simulink model "gm_sampleModel61753_pp_45_1_sub"  (R2023b)
settings: Solver=VariableStepAuto  StartTime=0.0  StopTime=10.0  RelTol=1e-3
libraries: simulink x43
(part 2 of 2)

== system gm_sampleModel61753_pp_45_1_sub/Subsystem/cfblk4 ==
  note: U(k)
  note: Edge
  U : Inport  OutDataTypeStr=uint8  SampleTime=1
  Delay Input1 : UnitDelay  Description=Store in Global RAM  DisableCoverage=on  InitialCondition=vinit  SampleTime=-1  HasFrameUpgradeWarning=on
  FixPt Relational Operator : RelationalOperator  Operator=>  OutDataTypeStr=fixdt(0, 8)  ZeroCross=off  InputSameDT=off
  Nonpositive : Subsystem  mask(Compare To Zero){relop=<=, OutDataTypeStr=boolean, ZeroCross=off}
      mask prompts: relop "Simulink:masks:Operator_MP"; OutDataTypeStr "Simulink:masks:OutputDataType_MP"; ZeroCross "Simulink:masks:EnableZerocrossingDetection_MP"
      mask help: Simulink:masks:CompareToZero_MD
      mask init:
      | OutDataTypeStr = 'boolean';
      | ZeroCross = 'off';
      | blkName = 'sampleModel61753_pp_45_1_sub/Subsystem/cfblk4/Nonpositive';
      | relop = '<=';
      | setValue = 'boolean';
      mask TypeOptions relop: == | ~= | < | <= | >= | >
      mask TypeOptions OutDataTypeStr: Simulink:masks:uint8 | Simulink:masks:boolean
      mask Callback ZeroCross: sl('zeroCrossEnable', gcbh);
      mask Display: disp([relop,' 0'])
  Y : Outport  SampleTime=1
  wires:
  U/1 -> Nonpositive/1(u)
  Delay Input1/1 -> FixPt Relational Operator/2
  FixPt Relational Operator/1 -> Y/1
  Nonpositive/1(y) -> FixPt Relational Operator/1, Delay Input1/1

== system gm_sampleModel61753_pp_45_1_sub/Subsystem/cfblk41 ==
  emi_236 : Inport  OutDataTypeStr=uint8  PortDimensions=1  SampleTime=1
  Action Port : Inport  Port=2  OutDataTypeStr=boolean  SampleTime=1
  cfblk41 : MinMax
  cfblk41_out1bypassMux : MultiPortSwitch  DataPortOrder=Zero-based contiguous  Inputs=2  zeroidx=on  OutDataTypeStr=uint8  SampleTime=1  SaturateOnIntegerOverflow=off  InputSameDT=off
  emi_237_bypass : UnitDelay  InitialCondition="fi(0,0,8,0,\"hex\",\"00\")"  SampleTime=1
  emi_237 : Outport  SampleTime=1  InitialOutput=0
  wires:
  Action Port/1 -> cfblk41_out1bypassMux/1
  emi_236/1 -> cfblk41/1
  cfblk41/1 -> cfblk41_out1bypassMux/3
  cfblk41_out1bypassMux/1 -> emi_237_bypass/1, emi_237/1
  emi_237_bypass/1 -> cfblk41_out1bypassMux/2

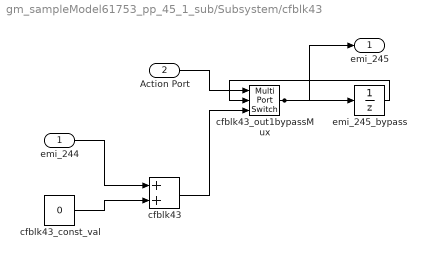
== system gm_sampleModel61753_pp_45_1_sub/Subsystem/cfblk43 ==
  emi_244 : Inport  OutDataTypeStr=uint8  PortDimensions=1  SampleTime=1
  Action Port : Inport  Port=2  OutDataTypeStr=boolean  SampleTime=1
  cfblk43 : Sum  OutDataTypeStr=uint8  AccumDataTypeStr=uint8  RndMeth=Nearest  SampleTime=1
  cfblk43_const_val : Constant  Value=0  VectorParams1D=off  OutDataTypeStr=uint8  SampleTime=1
  cfblk43_out1bypassMux : MultiPortSwitch  DataPortOrder=Zero-based contiguous  Inputs=2  zeroidx=on  OutDataTypeStr=uint8  SampleTime=1  SaturateOnIntegerOverflow=off  InputSameDT=off
  emi_245_bypass : UnitDelay  InitialCondition="fi(0,0,8,0,\"hex\",\"00\")"  SampleTime=1
  emi_245 : Outport  SampleTime=1  InitialOutput=0
  wires:
  Action Port/1 -> cfblk43_out1bypassMux/1
  emi_244/1 -> cfblk43/1
  cfblk43/1 -> cfblk43_out1bypassMux/3
  cfblk43_out1bypassMux/1 -> emi_245_bypass/1, emi_245/1
  emi_245_bypass/1 -> cfblk43_out1bypassMux/2
  cfblk43_const_val/1 -> cfblk43/2

== system gm_sampleModel61753_pp_45_1_sub/Subsystem/cfblk46 ==
  emi_252 : Inport  OutDataTypeStr=uint8  PortDimensions=1  SampleTime=1
  Action Port : Inport  Port=2  OutDataTypeStr=boolean  SampleTime=1
  cfblk46 : Sum  Inputs=+
  cfblk46_out1bypassMux : MultiPortSwitch  DataPortOrder=Zero-based contiguous  Inputs=2  zeroidx=on  OutDataTypeStr=uint8  SampleTime=1  SaturateOnIntegerOverflow=off  InputSameDT=off
  emi_253_bypass : UnitDelay  InitialCondition="fi(0,0,8,0,\"hex\",\"00\")"  SampleTime=1
  emi_253 : Outport  SampleTime=1  InitialOutput=0
  wires:
  Action Port/1 -> cfblk46_out1bypassMux/1
  emi_252/1 -> cfblk46/1
  cfblk46/1 -> cfblk46_out1bypassMux/3
  cfblk46_out1bypassMux/1 -> emi_253_bypass/1, emi_253/1
  emi_253_bypass/1 -> cfblk46_out1bypassMux/2

== system gm_sampleModel61753_pp_45_1_sub/Subsystem/cfblk48 ==
  emi_260 : Inport  OutDataTypeStr=uint8  PortDimensions=1  SampleTime=1
  Action Port : Inport  Port=2  OutDataTypeStr=boolean  SampleTime=1
  cfblk48 : Subsystem  mask(Real World Value Increment){}
      mask help: Simulink:masks:RealWorldValueIncrement_MD
      mask Display: disp('V++')
  cfblk48_out1bypassMux : MultiPortSwitch  DataPortOrder=Zero-based contiguous  Inputs=2  zeroidx=on  OutDataTypeStr=uint8  SampleTime=1  SaturateOnIntegerOverflow=off  InputSameDT=off
  emi_261_bypass : UnitDelay  InitialCondition="fi(0,0,8,0,\"hex\",\"00\")"  SampleTime=1
  emi_261 : Outport  SampleTime=1  InitialOutput=0
  wires:
  Action Port/1 -> cfblk48_out1bypassMux/1
  emi_260/1 -> cfblk48/1(u)
  cfblk48/1(y) -> cfblk48_out1bypassMux/3
  cfblk48_out1bypassMux/1 -> emi_261_bypass/1, emi_261/1
  emi_261_bypass/1 -> cfblk48_out1bypassMux/2

== system gm_sampleModel61753_pp_45_1_sub/Subsystem/cfblk50 ==
  emi_9 : Inport  OutDataTypeStr=uint8  PortDimensions=1  SampleTime=1
  Action Port : Inport  Port=2  OutDataTypeStr=boolean  SampleTime=1
  cfblk50 : Abs  SampleTime=1  OutDataTypeStr=uint8  SaturateOnIntegerOverflow=off
  cfblk50_out1bypassMux : MultiPortSwitch  DataPortOrder=Zero-based contiguous  Inputs=2  zeroidx=on  OutDataTypeStr=uint8  SampleTime=1  SaturateOnIntegerOverflow=off  InputSameDT=off
  emi_10_bypass : UnitDelay  InitialCondition="fi(0,0,8,0,\"hex\",\"00\")"  SampleTime=1
  emi_10 : Outport  SampleTime=1  InitialOutput=0
  wires:
  Action Port/1 -> cfblk50_out1bypassMux/1
  emi_9/1 -> cfblk50/1
  cfblk50/1 -> cfblk50_out1bypassMux/3
  cfblk50_out1bypassMux/1 -> emi_10_bypass/1, emi_10/1
  emi_10_bypass/1 -> cfblk50_out1bypassMux/2

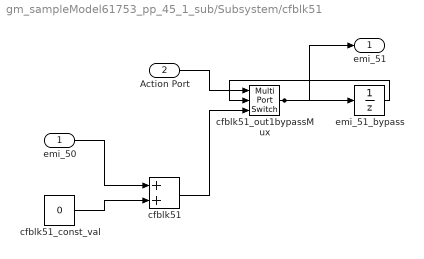
== system gm_sampleModel61753_pp_45_1_sub/Subsystem/cfblk51 ==
  emi_50 : Inport  OutDataTypeStr=uint8  PortDimensions=1  SampleTime=1
  Action Port : Inport  Port=2  OutDataTypeStr=boolean  SampleTime=1
  cfblk51 : Sum  OutDataTypeStr=uint8  AccumDataTypeStr=uint8  RndMeth=Nearest  SampleTime=1
  cfblk51_const_val : Constant  Value=0  VectorParams1D=off  OutDataTypeStr=uint8  SampleTime=1
  cfblk51_out1bypassMux : MultiPortSwitch  DataPortOrder=Zero-based contiguous  Inputs=2  zeroidx=on  OutDataTypeStr=uint8  SampleTime=1  SaturateOnIntegerOverflow=off  InputSameDT=off
  emi_51_bypass : UnitDelay  InitialCondition="fi(0,0,8,0,\"hex\",\"00\")"  SampleTime=1
  emi_51 : Outport  SampleTime=1  InitialOutput=0
  wires:
  Action Port/1 -> cfblk51_out1bypassMux/1
  emi_50/1 -> cfblk51/1
  cfblk51/1 -> cfblk51_out1bypassMux/3
  cfblk51_out1bypassMux/1 -> emi_51_bypass/1, emi_51/1
  emi_51_bypass/1 -> cfblk51_out1bypassMux/2
  cfblk51_const_val/1 -> cfblk51/2

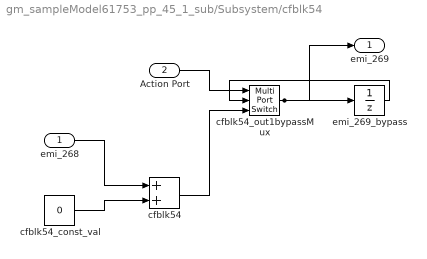
== system gm_sampleModel61753_pp_45_1_sub/Subsystem/cfblk54 ==
  emi_268 : Inport  OutDataTypeStr=uint8  PortDimensions=1  SampleTime=1
  Action Port : Inport  Port=2  OutDataTypeStr=boolean  SampleTime=1
  cfblk54 : Sum  OutDataTypeStr=uint8  AccumDataTypeStr=uint8  RndMeth=Nearest  SampleTime=1
  cfblk54_const_val : Constant  Value=0  VectorParams1D=off  OutDataTypeStr=uint8  SampleTime=1
  cfblk54_out1bypassMux : MultiPortSwitch  DataPortOrder=Zero-based contiguous  Inputs=2  zeroidx=on  OutDataTypeStr=uint8  SampleTime=1  SaturateOnIntegerOverflow=off  InputSameDT=off
  emi_269_bypass : UnitDelay  InitialCondition="fi(0,0,8,0,\"hex\",\"00\")"  SampleTime=1
  emi_269 : Outport  SampleTime=1  InitialOutput=0
  wires:
  Action Port/1 -> cfblk54_out1bypassMux/1
  emi_268/1 -> cfblk54/1
  cfblk54/1 -> cfblk54_out1bypassMux/3
  cfblk54_out1bypassMux/1 -> emi_269_bypass/1, emi_269/1
  emi_269_bypass/1 -> cfblk54_out1bypassMux/2
  cfblk54_const_val/1 -> cfblk54/2

== system gm_sampleModel61753_pp_45_1_sub/Subsystem/cfblk57 ==
  emi_276 : Inport  OutDataTypeStr=uint8  PortDimensions=1  SampleTime=1
  Action Port : Inport  Port=2  OutDataTypeStr=boolean  SampleTime=1
  cfblk57 : Signum  SampleTime=1
  cfblk57_out1bypassMux : MultiPortSwitch  DataPortOrder=Zero-based contiguous  Inputs=2  zeroidx=on  OutDataTypeStr=uint8  SampleTime=1  SaturateOnIntegerOverflow=off  InputSameDT=off
  emi_277_bypass : UnitDelay  InitialCondition="fi(0,0,8,0,\"hex\",\"00\")"  SampleTime=1
  emi_277 : Outport  SampleTime=1  InitialOutput=0
  wires:
  Action Port/1 -> cfblk57_out1bypassMux/1
  emi_276/1 -> cfblk57/1
  cfblk57/1 -> cfblk57_out1bypassMux/3
  cfblk57_out1bypassMux/1 -> emi_277_bypass/1, emi_277/1
  emi_277_bypass/1 -> cfblk57_out1bypassMux/2

== system gm_sampleModel61753_pp_45_1_sub/Subsystem/cfblk58 ==
  emi_284 : Inport  OutDataTypeStr=uint8  PortDimensions=1  SampleTime=1
  Action Port : Inport  Port=2  OutDataTypeStr=boolean  SampleTime=1
  cfblk58 : MinMax
  cfblk58_out1bypassMux : MultiPortSwitch  DataPortOrder=Zero-based contiguous  Inputs=2  zeroidx=on  OutDataTypeStr=uint8  SampleTime=1  SaturateOnIntegerOverflow=off  InputSameDT=off
  emi_285_bypass : UnitDelay  InitialCondition="fi(0,0,8,0,\"hex\",\"00\")"  SampleTime=1
  emi_285 : Outport  SampleTime=1  InitialOutput=0
  wires:
  Action Port/1 -> cfblk58_out1bypassMux/1
  emi_284/1 -> cfblk58/1
  cfblk58/1 -> cfblk58_out1bypassMux/3
  cfblk58_out1bypassMux/1 -> emi_285_bypass/1, emi_285/1
  emi_285_bypass/1 -> cfblk58_out1bypassMux/2

== system gm_sampleModel61753_pp_45_1_sub/Subsystem/cfblk62_inst ==
  in1 : Inport  OutDataTypeStr=uint8  SampleTime=1
  in2 : Inport  Port=2  OutDataTypeStr=uint8  SampleTime=1
  mul_cfblk62_dotp_mulcomp : Product  Inputs=**  OutDataTypeStr=uint8  SampleTime=1
  out1 : Outport  OutDataTypeStr=uint8  SampleTime=1
  wires:
  in1/1 -> mul_cfblk62_dotp_mulcomp/1
  in2/1 -> mul_cfblk62_dotp_mulcomp/2
  mul_cfblk62_dotp_mulcomp/1 -> out1/1

== system gm_sampleModel61753_pp_45_1_sub/Subsystem/cfblk65_inst ==
  in1 : Inport  OutDataTypeStr=uint8  SampleTime=1
  in2 : Inport  Port=2  OutDataTypeStr=uint8  SampleTime=1
  mul_cfblk65_dotp_mulcomp : Product  Inputs=**  OutDataTypeStr=uint8  SampleTime=1
  out1 : Outport  OutDataTypeStr=uint8  SampleTime=1
  wires:
  in1/1 -> mul_cfblk65_dotp_mulcomp/1
  in2/1 -> mul_cfblk65_dotp_mulcomp/2
  mul_cfblk65_dotp_mulcomp/1 -> out1/1

== system gm_sampleModel61753_pp_45_1_sub/Subsystem/cfblk69 ==
  emi_196 : Inport  OutDataTypeStr=uint8  PortDimensions=1  SampleTime=1
  Action Port : Inport  Port=2  OutDataTypeStr=boolean  SampleTime=1
  cfblk69 : Sum  Inputs=+
  cfblk69_out1bypassMux : MultiPortSwitch  DataPortOrder=Zero-based contiguous  Inputs=2  zeroidx=on  OutDataTypeStr=uint8  SampleTime=1  SaturateOnIntegerOverflow=off  InputSameDT=off
  emi_197_bypass : UnitDelay  InitialCondition="fi(0,0,8,0,\"hex\",\"00\")"  SampleTime=1
  emi_197 : Outport  SampleTime=1  InitialOutput=0
  wires:
  Action Port/1 -> cfblk69_out1bypassMux/1
  emi_196/1 -> cfblk69/1
  cfblk69/1 -> cfblk69_out1bypassMux/3
  cfblk69_out1bypassMux/1 -> emi_197_bypass/1, emi_197/1
  emi_197_bypass/1 -> cfblk69_out1bypassMux/2

== system gm_sampleModel61753_pp_45_1_sub/Subsystem/cfblk6_inst ==
  in1 : Inport  OutDataTypeStr=uint8  SampleTime=1
  in2 : Inport  Port=2  OutDataTypeStr=uint8  SampleTime=1
  mul_cfblk6_dotp_mulcomp : Product  Inputs=**  OutDataTypeStr=uint8  SampleTime=1
  out1 : Outport  OutDataTypeStr=uint8  SampleTime=1
  wires:
  in1/1 -> mul_cfblk6_dotp_mulcomp/1
  in2/1 -> mul_cfblk6_dotp_mulcomp/2
  mul_cfblk6_dotp_mulcomp/1 -> out1/1

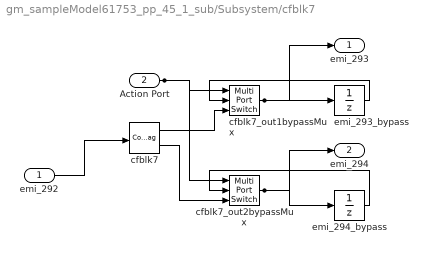
== system gm_sampleModel61753_pp_45_1_sub/Subsystem/cfblk7 ==
  emi_292 : Inport  OutDataTypeStr=uint8  PortDimensions=1  SampleTime=1
  Action Port : Inport  Port=2  OutDataTypeStr=boolean  SampleTime=1
  cfblk7 : ComplexToRealImag  SampleTime=1
  cfblk7_out1bypassMux : MultiPortSwitch  DataPortOrder=Zero-based contiguous  Inputs=2  zeroidx=on  OutDataTypeStr=uint8  SampleTime=1  SaturateOnIntegerOverflow=off  InputSameDT=off
  cfblk7_out2bypassMux : MultiPortSwitch  DataPortOrder=Zero-based contiguous  Inputs=2  zeroidx=on  OutDataTypeStr=uint8  SampleTime=1  SaturateOnIntegerOverflow=off  InputSameDT=off
  emi_293_bypass : UnitDelay  InitialCondition="fi(0,0,8,0,\"hex\",\"00\")"  SampleTime=1
  emi_294_bypass : UnitDelay  InitialCondition="fi(0,0,8,0,\"hex\",\"00\")"  SampleTime=1
  emi_293 : Outport  SampleTime=1  InitialOutput=0
  emi_294 : Outport  Port=2  SampleTime=1  InitialOutput=0
  wires:
  Action Port/1 -> cfblk7_out2bypassMux/1, cfblk7_out1bypassMux/1
  emi_292/1 -> cfblk7/1
  cfblk7/1 -> cfblk7_out1bypassMux/3
  cfblk7/2 -> cfblk7_out2bypassMux/3
  cfblk7_out1bypassMux/1 -> emi_293_bypass/1, emi_293/1
  emi_293_bypass/1 -> cfblk7_out1bypassMux/2
  cfblk7_out2bypassMux/1 -> emi_294_bypass/1, emi_294/1
  emi_294_bypass/1 -> cfblk7_out2bypassMux/2

== system gm_sampleModel61753_pp_45_1_sub/Subsystem/cfblk74_inst ==
  in1 : Inport  OutDataTypeStr=uint8  SampleTime=1
  in2 : Inport  Port=2  OutDataTypeStr=uint8  SampleTime=1
  mul_cfblk74_dotp_mulcomp : Product  Inputs=**  OutDataTypeStr=uint8  SampleTime=1
  out1 : Outport  OutDataTypeStr=uint8  SampleTime=1
  wires:
  in1/1 -> mul_cfblk74_dotp_mulcomp/1
  in2/1 -> mul_cfblk74_dotp_mulcomp/2
  mul_cfblk74_dotp_mulcomp/1 -> out1/1

== system gm_sampleModel61753_pp_45_1_sub/Subsystem/cfblk76 ==
  emi_301 : Inport  OutDataTypeStr=uint8  PortDimensions=1  SampleTime=1
  Action Port : Inport  Port=2  OutDataTypeStr=boolean  SampleTime=1
  cfblk76 : Gain  Gain="fi(0,0,8,7,\"hex\",\"80\")"  ParamDataTypeStr=fixdt(0, 8, 7)  OutDataTypeStr=fixdt(0, 16, 7)  SampleTime=1
  cfblk76_out1bypassMux : MultiPortSwitch  DataPortOrder=Zero-based contiguous  Inputs=2  zeroidx=on  OutDataTypeStr=fixdt(0, 16, 7)  SampleTime=1  SaturateOnIntegerOverflow=off  InputSameDT=off
  emi_302_bypass : UnitDelay  InitialCondition="fi(0,0,16,7,\"hex\",\"0000\")"  SampleTime=1
  emi_302 : Outport  SampleTime=1  InitialOutput=0
  wires:
  Action Port/1 -> cfblk76_out1bypassMux/1
  emi_301/1 -> cfblk76/1
  cfblk76/1 -> cfblk76_out1bypassMux/3
  cfblk76_out1bypassMux/1 -> emi_302_bypass/1, emi_302/1
  emi_302_bypass/1 -> cfblk76_out1bypassMux/2

== system gm_sampleModel61753_pp_45_1_sub/Subsystem/cfblk83_inst ==
  in1 : Inport  OutDataTypeStr=uint8  SampleTime=1
  in2 : Inport  Port=2  OutDataTypeStr=uint8  SampleTime=1
  mul_cfblk83_dotp_mulcomp : Product  Inputs=**  OutDataTypeStr=uint8  SampleTime=1
  out1 : Outport  OutDataTypeStr=uint8  SampleTime=1
  wires:
  in1/1 -> mul_cfblk83_dotp_mulcomp/1
  in2/1 -> mul_cfblk83_dotp_mulcomp/2
  mul_cfblk83_dotp_mulcomp/1 -> out1/1

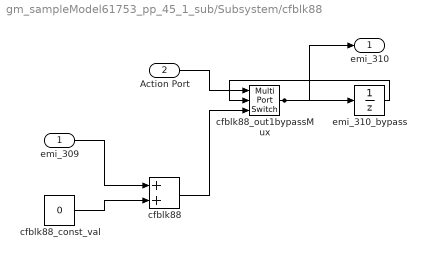
== system gm_sampleModel61753_pp_45_1_sub/Subsystem/cfblk88 ==
  emi_309 : Inport  OutDataTypeStr=uint8  PortDimensions=1  SampleTime=1
  Action Port : Inport  Port=2  OutDataTypeStr=boolean  SampleTime=1
  cfblk88 : Sum  OutDataTypeStr=uint8  AccumDataTypeStr=uint8  RndMeth=Nearest  SampleTime=1
  cfblk88_const_val : Constant  Value=0  VectorParams1D=off  OutDataTypeStr=uint8  SampleTime=1
  cfblk88_out1bypassMux : MultiPortSwitch  DataPortOrder=Zero-based contiguous  Inputs=2  zeroidx=on  OutDataTypeStr=uint8  SampleTime=1  SaturateOnIntegerOverflow=off  InputSameDT=off
  emi_310_bypass : UnitDelay  InitialCondition="fi(0,0,8,0,\"hex\",\"00\")"  SampleTime=1
  emi_310 : Outport  SampleTime=1  InitialOutput=0
  wires:
  Action Port/1 -> cfblk88_out1bypassMux/1
  emi_309/1 -> cfblk88/1
  cfblk88/1 -> cfblk88_out1bypassMux/3
  cfblk88_out1bypassMux/1 -> emi_310_bypass/1, emi_310/1
  emi_310_bypass/1 -> cfblk88_out1bypassMux/2
  cfblk88_const_val/1 -> cfblk88/2

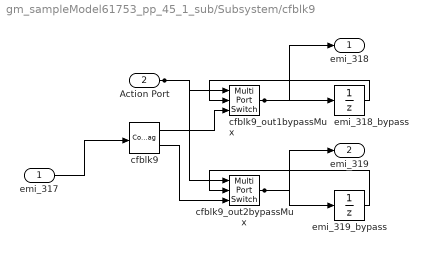
== system gm_sampleModel61753_pp_45_1_sub/Subsystem/cfblk9 ==
  emi_317 : Inport  OutDataTypeStr=uint8  PortDimensions=1  SampleTime=1
  Action Port : Inport  Port=2  OutDataTypeStr=boolean  SampleTime=1
  cfblk9 : ComplexToRealImag  SampleTime=1
  cfblk9_out1bypassMux : MultiPortSwitch  DataPortOrder=Zero-based contiguous  Inputs=2  zeroidx=on  OutDataTypeStr=uint8  SampleTime=1  SaturateOnIntegerOverflow=off  InputSameDT=off
  cfblk9_out2bypassMux : MultiPortSwitch  DataPortOrder=Zero-based contiguous  Inputs=2  zeroidx=on  OutDataTypeStr=uint8  SampleTime=1  SaturateOnIntegerOverflow=off  InputSameDT=off
  emi_318_bypass : UnitDelay  InitialCondition="fi(0,0,8,0,\"hex\",\"00\")"  SampleTime=1
  emi_319_bypass : UnitDelay  InitialCondition="fi(0,0,8,0,\"hex\",\"00\")"  SampleTime=1
  emi_318 : Outport  SampleTime=1  InitialOutput=0
  emi_319 : Outport  Port=2  SampleTime=1  InitialOutput=0
  wires:
  Action Port/1 -> cfblk9_out2bypassMux/1, cfblk9_out1bypassMux/1
  emi_317/1 -> cfblk9/1
  cfblk9/1 -> cfblk9_out1bypassMux/3
  cfblk9/2 -> cfblk9_out2bypassMux/3
  cfblk9_out1bypassMux/1 -> emi_318_bypass/1, emi_318/1
  emi_318_bypass/1 -> cfblk9_out1bypassMux/2
  cfblk9_out2bypassMux/1 -> emi_319_bypass/1, emi_319/1
  emi_319_bypass/1 -> cfblk9_out2bypassMux/2

== system gm_sampleModel61753_pp_45_1_sub/Subsystem/cfblk93 ==
  emi_326 : Inport  OutDataTypeStr=uint8  PortDimensions=1  SampleTime=1
  Action Port : Inport  Port=2  OutDataTypeStr=boolean  SampleTime=1
  Reshape : Reshape
  cfblk93_out1bypassMux : MultiPortSwitch  DataPortOrder=Zero-based contiguous  Inputs=2  zeroidx=on  OutDataTypeStr=uint8  SampleTime=1  SaturateOnIntegerOverflow=off  InputSameDT=off
  emi_327_bypass : UnitDelay  InitialCondition="fi(0,0,8,0,\"hex\",\"00\")"  SampleTime=1
  emi_327 : Outport  SampleTime=1  InitialOutput=0
  wires:
  Action Port/1 -> cfblk93_out1bypassMux/1
  emi_326/1 -> Reshape/1
  Reshape/1 -> cfblk93_out1bypassMux/3
  cfblk93_out1bypassMux/1 -> emi_327_bypass/1, emi_327/1
  emi_327_bypass/1 -> cfblk93_out1bypassMux/2

== system gm_sampleModel61753_pp_45_1_sub/Subsystem/cfblk95 ==
  emi_334 : Inport  OutDataTypeStr=uint8  PortDimensions=1  SampleTime=1
  Action Port : Inport  Port=2  OutDataTypeStr=boolean  SampleTime=1
  cfblk95 : Sum  OutDataTypeStr=uint8  AccumDataTypeStr=uint8  RndMeth=Nearest  SampleTime=1
  cfblk95_const_val : Constant  Value=0  VectorParams1D=off  OutDataTypeStr=uint8  SampleTime=1
  cfblk95_out1bypassMux : MultiPortSwitch  DataPortOrder=Zero-based contiguous  Inputs=2  zeroidx=on  OutDataTypeStr=uint8  SampleTime=1  SaturateOnIntegerOverflow=off  InputSameDT=off
  emi_335_bypass : UnitDelay  InitialCondition="fi(0,0,8,0,\"hex\",\"00\")"  SampleTime=1
  emi_335 : Outport  SampleTime=1  InitialOutput=0
  wires:
  Action Port/1 -> cfblk95_out1bypassMux/1
  emi_334/1 -> cfblk95/1
  cfblk95/1 -> cfblk95_out1bypassMux/3
  cfblk95_out1bypassMux/1 -> emi_335_bypass/1, emi_335/1
  emi_335_bypass/1 -> cfblk95_out1bypassMux/2
  cfblk95_const_val/1 -> cfblk95/2

== system gm_sampleModel61753_pp_45_1_sub/Subsystem/cfblk97 ==
  emi_342 : Inport  OutDataTypeStr=uint8  PortDimensions=1  SampleTime=1
  Action Port : Inport  Port=2  OutDataTypeStr=boolean  SampleTime=1
  cfblk97 : Subsystem  mask(Real World Value Increment){}
      mask help: Simulink:masks:RealWorldValueIncrement_MD
      mask Display: disp('V++')
  cfblk97_out1bypassMux : MultiPortSwitch  DataPortOrder=Zero-based contiguous  Inputs=2  zeroidx=on  OutDataTypeStr=uint8  SampleTime=1  SaturateOnIntegerOverflow=off  InputSameDT=off
  emi_343_bypass : UnitDelay  InitialCondition="fi(0,0,8,0,\"hex\",\"00\")"  SampleTime=1
  emi_343 : Outport  SampleTime=1  InitialOutput=0
  wires:
  Action Port/1 -> cfblk97_out1bypassMux/1
  emi_342/1 -> cfblk97/1(u)
  cfblk97/1(y) -> cfblk97_out1bypassMux/3
  cfblk97_out1bypassMux/1 -> emi_343_bypass/1, emi_343/1
  emi_343_bypass/1 -> cfblk97_out1bypassMux/2

== system gm_sampleModel61753_pp_45_1_sub/Subsystem/cfblk1/cfblk1 ==
  note: U(k)
  note: Edge
  U : Inport  OutDataTypeStr=uint8  SampleTime=1
  Action Port_out2 : Inport  Port=2  OutDataTypeStr=boolean  SampleTime=1
  Delay Input1 : Subsystem
      settings: MinAlgLoopOccurrences=on
  FixPt Relational Operator : RelationalOperator  Operator=>  OutDataTypeStr=fixdt(0,8,0)  SampleTime=1  InputSameDT=off
  Nonnegative : Subsystem  mask(Compare To Zero){relop=>=, OutDataTypeStr=boolean, ZeroCross=off}
      mask prompts: relop "Simulink:masks:Operator_MP"; OutDataTypeStr "Simulink:masks:OutputDataType_MP"; ZeroCross "Simulink:masks:EnableZerocrossingDetection_MP"
      mask help: Simulink:masks:CompareToZero_MD
      mask TypeOptions relop: == | ~= | < | <= | >= | >
      mask TypeOptions OutDataTypeStr: Simulink:masks:uint8 | Simulink:masks:boolean
      mask Callback ZeroCross: sl('zeroCrossEnable', gcbh);
      mask Display: disp([relop,' 0'])
  Y : Outport  SampleTime=1  InitialOutput=0
  wires:
  U/1 -> Nonnegative/1(u)
  Delay Input1/1(out0) -> FixPt Relational Operator/2
  FixPt Relational Operator/1 -> Y/1
  Nonnegative/1(y) -> FixPt Relational Operator/1, Delay Input1/1(in0)
  Action Port_out2/1 -> Delay Input1/Enable

== system gm_sampleModel61753_pp_45_1_sub/Subsystem/cfblk150/cfblk150 ==
  u : Inport  OutDataTypeStr=uint8  SampleTime=1
  FixPt Constant : Constant  DisableCoverage=on  OutDataTypeStr=Inherit: Inherit via back propagation  SampleTime=-1
  FixPt Data Type Duplicate : DataTypeDuplicate  DisableCoverage=on  NumInputPorts=3
  FixPt Sum1 : Sum  OutDataTypeStr=Inherit: Inherit via back propagation  InputSameDT=on  LockScale=on
  y : Outport  SampleTime=1  InitialOutput=0
  wires:
  u/1 -> FixPt Sum1/1, FixPt Data Type Duplicate/2
  FixPt Constant/1 -> FixPt Sum1/2, FixPt Data Type Duplicate/3
  FixPt Sum1/1 -> FixPt Data Type Duplicate/1, y/1

== system gm_sampleModel61753_pp_45_1_sub/Subsystem/cfblk159/cfblk159 ==
  In1 : Inport  OutDataTypeStr=uint8  PortDimensions=1  SampleTime=1
  Out1 : Outport  SampleTime=1  InitialOutput=0
  wires:
  In1/1 -> Out1/1

== system gm_sampleModel61753_pp_45_1_sub/Subsystem/cfblk165/cfblk165 ==
  in0 : Inport  OutDataTypeStr=uint8  SampleTime=1
  Action Port_out2 : EnablePort  OutDataTypeStr=boolean
  cfblk165 : Delay  DelayLength=double(2)  InitialCondition=0
  out0 : Outport  OutDataTypeStr=uint8  SampleTime=1  InitialOutput=0
  wires:
  cfblk165/1 -> out0/1
  in0/1 -> cfblk165/1

== system gm_sampleModel61753_pp_45_1_sub/Subsystem/cfblk167/cfblk167 ==
  in0 : Inport  OutDataTypeStr=uint8  SampleTime=1
  Action Port_out2 : EnablePort  OutDataTypeStr=boolean
  cfblk167 : Delay  DelayLength=double(2)  InitialCondition=0
  out0 : Outport  OutDataTypeStr=uint8  SampleTime=1  InitialOutput=0
  wires:
  cfblk167/1 -> out0/1
  in0/1 -> cfblk167/1

== system gm_sampleModel61753_pp_45_1_sub/Subsystem/cfblk172/cfblk172 ==
  in0 : Inport  OutDataTypeStr=uint8  SampleTime=1
  Action Port_out2 : EnablePort  OutDataTypeStr=boolean
  cfblk172 : Delay  DelayLength=double(2)  InitialCondition=0
  out0 : Outport  OutDataTypeStr=uint8  SampleTime=1  InitialOutput=0
  wires:
  cfblk172/1 -> out0/1
  in0/1 -> cfblk172/1

== system gm_sampleModel61753_pp_45_1_sub/Subsystem/cfblk2/Positive ==
  u : Inport  OutDataTypeStr=uint8  SampleTime=1
  Compare : RelationalOperator  Operator=>  OutDataTypeStr=boolean  ZeroCross=off
  Constant : Constant  DisableCoverage=on  Value=0  OutDataTypeStr=Inherit: Inherit via back propagation  SampleTime=-1  PreserveConstantTs=on
  y : Outport  SampleTime=1
  wires:
  u/1 -> Compare/1
  Compare/1 -> y/1
  Constant/1 -> Compare/2

== system gm_sampleModel61753_pp_45_1_sub/Subsystem/cfblk3/Nonnegative ==
  u : Inport  OutDataTypeStr=uint8  SampleTime=1
  Compare : RelationalOperator  OutDataTypeStr=boolean  ZeroCross=off
  Constant : Constant  DisableCoverage=on  Value=0  OutDataTypeStr=Inherit: Inherit via back propagation  SampleTime=-1  PreserveConstantTs=on
  y : Outport  SampleTime=1
  wires:
  u/1 -> Compare/1
  Compare/1 -> y/1
  Constant/1 -> Compare/2

== system gm_sampleModel61753_pp_45_1_sub/Subsystem/cfblk30/cfblk30 ==
  u : Inport  OutDataTypeStr=uint8  SampleTime=1
  FixPt Constant : Constant  DisableCoverage=on  OutDataTypeStr=Inherit: Inherit via back propagation  SampleTime=-1
  FixPt Data Type Duplicate : DataTypeDuplicate  DisableCoverage=on  NumInputPorts=3
  FixPt Sum1 : Sum  OutDataTypeStr=Inherit: Inherit via back propagation  InputSameDT=on  LockScale=on
  y : Outport  SampleTime=1  InitialOutput=0
  wires:
  u/1 -> FixPt Sum1/1, FixPt Data Type Duplicate/2
  FixPt Constant/1 -> FixPt Sum1/2, FixPt Data Type Duplicate/3
  FixPt Sum1/1 -> FixPt Data Type Duplicate/1, y/1

== system gm_sampleModel61753_pp_45_1_sub/Subsystem/cfblk4/Nonpositive ==
  u : Inport  OutDataTypeStr=uint8  SampleTime=1
  Compare : RelationalOperator  Operator=<=  OutDataTypeStr=boolean  ZeroCross=off
  Constant : Constant  DisableCoverage=on  Value=0  OutDataTypeStr=Inherit: Inherit via back propagation  SampleTime=-1  PreserveConstantTs=on
  y : Outport  SampleTime=1
  wires:
  u/1 -> Compare/1
  Compare/1 -> y/1
  Constant/1 -> Compare/2

== system gm_sampleModel61753_pp_45_1_sub/Subsystem/cfblk48/cfblk48 ==
  u : Inport  OutDataTypeStr=uint8  SampleTime=1
  FixPt Constant : Constant  DisableCoverage=on  OutDataTypeStr=Inherit: Inherit via back propagation  SampleTime=-1
  FixPt Data Type Duplicate : DataTypeDuplicate  DisableCoverage=on  NumInputPorts=3
  FixPt Sum1 : Sum  OutDataTypeStr=Inherit: Inherit via back propagation  InputSameDT=on  LockScale=on
  y : Outport  SampleTime=1  InitialOutput=0
  wires:
  u/1 -> FixPt Sum1/1, FixPt Data Type Duplicate/2
  FixPt Constant/1 -> FixPt Sum1/2, FixPt Data Type Duplicate/3
  FixPt Sum1/1 -> FixPt Data Type Duplicate/1, y/1

== system gm_sampleModel61753_pp_45_1_sub/Subsystem/cfblk97/cfblk97 ==
  u : Inport  OutDataTypeStr=uint8  SampleTime=1
  FixPt Constant : Constant  DisableCoverage=on  OutDataTypeStr=Inherit: Inherit via back propagation  SampleTime=-1
  FixPt Data Type Duplicate : DataTypeDuplicate  DisableCoverage=on  NumInputPorts=3
  FixPt Sum1 : Sum  OutDataTypeStr=Inherit: Inherit via back propagation  InputSameDT=on  LockScale=on
  y : Outport  SampleTime=1  InitialOutput=0
  wires:
  u/1 -> FixPt Sum1/1, FixPt Data Type Duplicate/2
  FixPt Constant/1 -> FixPt Sum1/2, FixPt Data Type Duplicate/3
  FixPt Sum1/1 -> FixPt Data Type Duplicate/1, y/1

== system gm_sampleModel61753_pp_45_1_sub/Subsystem/cfblk1/cfblk1/Delay Input1 ==
  in0 : Inport  OutDataTypeStr=boolean  SampleTime=1
  Action Port_out2 : EnablePort  OutDataTypeStr=boolean
  Delay Input1 : UnitDelay  SampleTime=1
  out0 : Outport  OutDataTypeStr=boolean  SampleTime=1  InitialOutput=0
  wires:
  Delay Input1/1 -> out0/1
  in0/1 -> Delay Input1/1

== system gm_sampleModel61753_pp_45_1_sub/Subsystem/cfblk1/cfblk1/Nonnegative ==
  u : Inport  OutDataTypeStr=uint8  SampleTime=1
  Compare : RelationalOperator  OutDataTypeStr=boolean  SampleTime=1
  Constant : Constant  Value=0  OutDataTypeStr=uint8  SampleTime=1
  y : Outport  SampleTime=1  InitialOutput=0
  wires:
  u/1 -> Compare/1
  Compare/1 -> y/1
  Constant/1 -> Compare/2
